simulink model "DynamicMemoryAllocationTest"  (R2022a)
settings: Solver=FixedStepAuto  StartTime=0.0  StopTime=10.0  RelTol=1e-3
libraries: visiontransforms x1
settings Model: Creator=jinch  LastModifiedBy=jinch

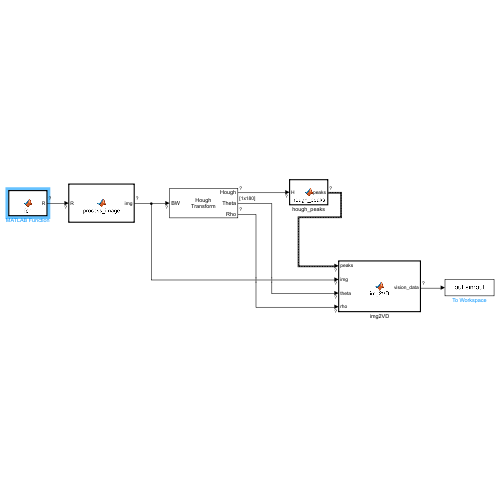
[thumbnail: Simulink's stored preview of the top-level diagram]
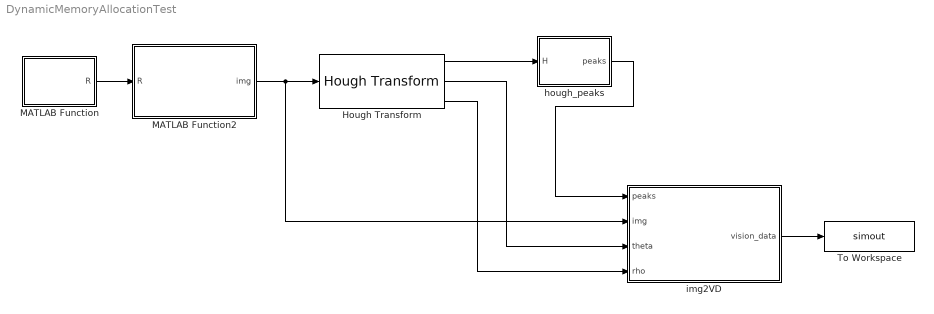
== system DynamicMemoryAllocationTest ==
  Hough Transform : visiontransforms/Hough Transform  theta_res=pi/180  rho_res=1  out_theta_rho=on  outdtmode=double  roundingMode=Nearest  overflowMode=on  firstCoeffMode=Binary point scaling  firstCoeffWordLength=16  firstCoeffFracLength=14  secondCoeffMode=Binary point scaling  secondCoeffWordLength=32  secondCoeffFracLength=16  prodOutputMode=Binary point scaling  prodOutputWordLength=32  prodOutputFracLength=20  accumMode=Binary point scaling  accumWordLength=32  accumFracLength=20  outputMode=Binary point scaling  outputWordLength=16  outputFracLength=0  memoryMode=Binary point scaling  memoryWordLength=32  memoryFracLength=16
      settings: SourceProductBaseCode=VP
  MATLAB Function : MATLAB Function  TreatAsAtomicUnit=on
  MATLAB Function2 : MATLAB Function  TreatAsAtomicUnit=on
  To Workspace : ToWorkspace  VariableName=simout  SaveFormat=Timeseries  SampleTime=-1
  hough_peaks : MATLAB Function  TreatAsAtomicUnit=on
  img2VD : MATLAB Function  TreatAsAtomicUnit=on
  wires:
  Hough Transform/1 -> hough_peaks/1(H)
  Hough Transform/2 -> img2VD/3(theta)
  hough_peaks/1(peaks) -> img2VD/1(peaks)
  Hough Transform/3 -> img2VD/4(rho)
  MATLAB Function2/1(img) -> img2VD/2(img), Hough Transform/1
  MATLAB Function/1(R) -> MATLAB Function2/1(R)
  img2VD/1(vision_data) -> To Workspace/1

== matlab function DynamicMemoryAllocationTest/MATLAB Function ==
  data: R output
function R = fcn()
    R=cast(zeros(120, 160),"uint8");
    img = imread("test.jpg");
    R = img(:,:,1);
end

== matlab function DynamicMemoryAllocationTest/hough_peaks ==
  data: H input; peaks output size=[10 2]
function peaks = hough_peaks(H)
    peaks = houghpeaks(H,10,"NHoodSize",[13,13]);
end

== matlab function DynamicMemoryAllocationTest/MATLAB Function2 ==
  data: R input; img output
function img = process_image(R)

    redBW = imbinarize(R); % remove background if needed
    % redBW3 = bwskel(redBW); % doesn't work well due to branched endpoints
    redBW2 = bwmorph(redBW,"thin",6); % num of operations to be adjusted, edges to be solved
    redBW3 = bwmorph(redBW2,"skeleton",3);
    img = redBW3;

end

== matlab function DynamicMemoryAllocationTest/img2VD ==
  data: peaks input; img input; vision_data output size=[3 11]; theta input; rho input
function vision_data = img2VD(peaks, img,theta,rho)
    
    lines = houghlines(img,theta,rho,peaks);

    % set up
    vision_data = zeros([3 11]);
    vision_data(3,:) = -1;

    points = lines;
    counter_edge=0;
    
    for i = 1:length(lines)
        xy = [lines(i).point1; lines(i).point2];
        [row,~] = find((xy<10)+(xy(:,1)>150)+(xy(:,2)>110));
        if ~isempty(row)
            % finding points at the edge
            if row == 1
                points(i).point1(3)=1;
                counter_edge = counter_edge + 1;
                    if counter_edge == 1 
                        vision_data(:,1) = transpose(points(i).point1);
                        starting_line_number = i;
                        starting_point_number = 0; % 0 means point1; 1 means point 2
                    end
            end
    
            if row == 2
                points(i).point2(3)=1;
                counter_edge = counter_edge + 1;
                    if counter_edge == 1 
                        vision_data(:,1) = transpose(points(i).point2);
                        starting_line_number = 1;
                    end
            end      
        end
    end
    
    % Label and arrange section points
    points = struct2cell(points);
    second_point = points{~starting_point_number+1,1,starting_line_number};
    counter = 1;
    
    while length(points) >= 1 && ~isempty(second_point)
    
        for i = 1:length(points(1,1,:)) % length won't change even after deleting one line
            point1 = points{1,1,i};
            point2 = points{2,1,i};
            distance1 = sqrt((point1(1)-second_point(1))^2 + (point1(2)-second_point(2))^2);
            distance2 = sqrt((point2(1)-second_point(1))^2 + (point2(2)-second_point(2))^2);
        
            if distance1 < 8
                counter = counter+1;
                points{1,1,i}(3) = 0;
                vision_data(:,counter) = transpose(points{1,1,i});
                second_point = points{2,1,i};
                points(:,:,i) = [];
                if length(points(1,1,:))==1 && length(lines) ~= 1 % in case there's only one line
                    second_point(3) = 2;
                    vision_data(:,counter+1) = transpose(second_point);
                    points(:,:,i) = [];
                end
                break
                
    
            elseif distance2 < 8
                counter = counter+1;
                points{2,1,i}(3) = 0;
                vision_data(:,counter) = transpose(points{2,1,i});
                second_point = points{1,1,i};
                points(:,:,i) = [];
                if length(points(1,1,:))==1 && length(lines) ~= 1 % in case there's only one line
                    second_point(3) = 2;
                    vision_data(:,counter+1) = transpose(second_point);
                    points(:,:,i) = [];
                end
                break
            end  
        end
    end
    


    % Find circular landing point (assume only one)
    [c,~] = imfindcircles(R, [10 25]);
    if ~isempty(c)
        c(3) = 3;
        vision_data(:,counter+2) = transpose(c);
    end



end
